simulink library "vmc"  (R2021b)
settings: Solver=VariableStepAuto  StartTime=0.0  StopTime=10.0  RelTol=1e-3
undefined symbols (not defined in the file or in its folder): AVMC_ACCDeltaTqIGain4OVRD_X_kph, AVMC_ACCDeltaTqIGain4OVRD_Y_mps2, AVMC_ACCDeltaTqIGain_X_kph, AVMC_ACCDeltaTqIGain_Y_mps2, AVMC_ACCDeltaTqPGain_X_kph, AVMC_ACCDeltaTqPGain_Y_kph, AVMC_ACCLongSteadyCtrl_X_kph, AVMC_ADSPosGFBDeltaTq_X_kph, AVMC_ADSPosGFBDeltaTq_Y_mps2, AVMC_AggressJerkPCT4AT_X_kph, AVMC_AggressJerkPCT_X_kph, AVMC_AggressLimitPCT4AT_X_kph, AVMC_AggressLimitPCT_X_kph, AVMC_CCLongSteadyCtrl_X_kph, AVMC_DISCDeltaTqIGain_X_kph, AVMC_DISCDeltaTqIGain_Y_mps2, AVMC_DISCDeltaTqPGain_X_kph, AVMC_DISCDeltaTqPGain_Y_kph, AVMC_ESCRegenOut_X_kph, AVMC_ESCRegenOut_Y_Deg, AVMC_ESCRegenOutEnSpd_X_Deg, AVMC_ISOAccLimit_X_mps, AVMC_ISODecLimit_X_mps, AVMC_ISOJerk_X_mps, AVMC_LatESCRegenOut_X_kph, AVMC_LatESCRegenOut_Y_Deg, AVMC_LongAccDeadZone_X_kph, AVMC_LongAccFiltTsforP2_X_Gps, AVMC_MCPresBaseTq_X_bar, AVMC_MSALongSteadyCtrl_X_kph, AVMC_MSAPedalOvrd_X_kph, AVMC_MSASpdBand_X_kph, AVMC_MSATqDownEndTq_X_kph, AVMC_MSATqDownTime_X_kph, AVMC_OPDDisSlideRate_X_Deg, AVMC_OVRD2ActSR2FCMCMD_X_mps2, AVMC_PedalTqRWhlRatio_X_Nm, AVMC_PedalTqRWhlRatio_Y_gps, AVMC_PedalTqRWhlSlipGain_X_rat, AVMC_PedalTqRWhlSlipGain_Y_kph, AVMC_PedalTqRWhSTRGGain_X_deg, AVMC_PedalTqRWhSTRGGain_Y_kph, AVMC_RDCDetectTime_X_kph, AVMC_RDCDetectTime_Y_pct, AVMC_RDCEnSlideRate_X_Deg, AVMC_RearWhlTqRatio_X_Nm, AVMC_RearWhlTqRatio_Y_gps, AVMC_RearWhlTqSlipGain_X_rat, AVMC_RearWhlTqSlipGain_Y_kph, AVMC_RearWhlTqSTRGGain_X_deg, AVMC_RearWhlTqSTRGGain_Y_kph, AVMC_ReqBrkJoinDecSR_X_mps2, AVMC_SoftJerkPCT_X_kph, AVMC_SoftLimitPCT_X_kph, AVMC_StESCYaw_X_kph, AVMC_StESCYaw_Y_Deg, AVMC_StESCYawCom_X_kph, AVMC_StESCYawCom_Y_Gps, AVMC_TMSpdBaseTq_X_rpm, AVMC_VehHoldDecCtrlTime2_X_kph ... (+405)
libraries: hcu_lib x105, simulink x75, tqr x1, simulink_extras x1
(part 13 of 14)

== system vmc/VMC/VMC/Slide Rate  Calculation/4Wheel Calculation/RR Wheel ==
  VVMC_4WheelLongAcc_Gps : Inport
  task_time_s : Inport  Port=2
  VINP_RRRawWhlSpeed_kph : Inport  Port=3
  VTQD_GearActualPosn_enum : Inport  Port=4
  AND4 : Logic  Inputs=3  AllPortsSameDT=off  OutDataTypeStr=boolean
  Abs3 : Abs
  Add : Sum
  Add{3,8,15..16} (4 alike) : Sum  Inputs=+-
  Constant1 : Constant  Value=GRAVITY_G
  Constant11 : Constant  Value=KPH2MPS
  Constant14 : Constant  Value=ONE_PERCENT
  Constant15 : Constant  Value=KVMC_RawWhlSpeedDeadZone_kph
  Constant16 : Constant  Value=ZERO_FLOAT
  Constant17 : Constant  Value=KVMC_RawWhlSpeedDeadZone_kph
  Constant18 : Constant  Value=ONE_FLOAT
  Constant2 : Constant  Value=MPS2KPH
  Constant33 : Constant  Value=KPH2MPS
  Constant34 : Constant  Value=GRAVITY_G
  Constant35 : Constant  Value=KVMC_WhlSpdCalAccTs_c
  Constant42 : Constant  Value=KVMC_WheelSkidAccDev_Gps
  Constant43 : Constant  Value=KVMC_SkidRecVehSpdDev_kph
  Constant44 : Constant  Value=KPH2MPS
  Constant46 : Constant  Value=ENUM_GEARACTUALPOSN_D
  Constant47 : Constant  Value=ENUM_GEARACTUALPOSN_R
  Constant48 : Constant  Value=KVMC_PreVehSpdCalSW_flg
  Constant49 : Constant  Value=KVMC_RRWhlSkidReset_flg
  Constant5 : Constant  Value=KVMC_4WheelEnSkidDetSpd_kph
  Delay{,4..5,12..13,17} (6 alike) : Delay  DelayLength=1
  Divide3 : Product  Inputs=*//
  Divide7 : Product  Inputs=**//
  Equal : RelationalOperator  Operator===  OutDataTypeStr=boolean  RndMeth=Simplest
  Equal1 : RelationalOperator  Operator===  OutDataTypeStr=boolean  RndMeth=Simplest
  FirstOrderFilter3 : hcu_lib/Basic_Blocks/FirstOrderFilter
  OR : Logic  Operator=OR  AllPortsSameDT=off  OutDataTypeStr=boolean
  OR1 : Logic  Operator=OR  AllPortsSameDT=off  OutDataTypeStr=boolean
  OR2 : Logic  Operator=OR  AllPortsSameDT=off  OutDataTypeStr=boolean
  Product : Product
  Product1 : Product  Inputs=3
  Product2 : Product
  Product3 : Product
  Relational Operator14 : RelationalOperator  Operator=>  OutDataTypeStr=boolean  RndMeth=Simplest
  Relational Operator{2,5..6,15} (4 alike) : RelationalOperator  Operator=<=  OutDataTypeStr=boolean  RndMeth=Simplest
  SR_Latch3 : hcu_lib/Basic_Blocks/SR_Latch
  Saturation : Saturate  UpperLimit=KVMC_PredVehSpdLimit_mps  LowerLimit=ZERO_FLOAT
  Switch{,5..6,10} (4 alike) : Switch  Criteria=u2 > Threshold
  VVMC_RRPreVehSpd_kph : Outport
  VVMC_RRWhlSkid_flg : Outport  Port=2
  VVMC_RR4WhlSpdSlideRate_pct : Outport  Port=3
  wires:
  [VINP_RRRawWhlSpeed_kph] -> Add8/1
  Constant49/1 -> AND4/3
  Add8/1 -> Divide7/1
  [task_time_s] -> Divide7/3
  Add15/1 -> Abs3/1
  Relational Operator14/1 -> SR_Latch3/1
  [VVMC_4WheelLongAcc_Gps] -> Add16/2
  [task_time_s] -> FirstOrderFilter3/2
  [VINP_RRRawWhlSpeed_kph] -> Delay4/1
  Constant42/1 -> Relational Operator14/2
  FirstOrderFilter3/1 -> [VVMC_RRWhlCalAcc_Gps]  "VVMC_RRWhlCalAcc_Gps"
  Divide7/1 -> FirstOrderFilter3/1
  Relational Operator15/1 -> AND4/1
  Delay4/1 -> Add8/2
  Delay17/1 -> AND4/2
  [VVMC_RRWhlSkid_flg] -> Delay17/1
  Add16/1 -> Relational Operator14/1
  Delay12/1 -> Add15/1
  Constant43/1 -> Relational Operator15/2
  Delay13/1 -> Add15/2
  Constant33/1 -> Divide7/2
  Constant34/1 -> Divide7/4
  Abs3/1 -> Relational Operator15/1
  SR_Latch3/1 -> [VVMC_RRWhlSkid_flg]  "VVMC_RRWhlSkid_flg"
  [VVMC_RRWhlCalAcc_Gps] -> Add16/1
  Constant35/1 -> FirstOrderFilter3/3
  Constant14/1 -> Divide3/2
  Switch5/1 -> Divide3/3
  Divide3/1 -> Switch6/3  "VVMC_RRCal4WhlSpdSlideRate_pct"
  Switch6/1 -> [VVMC_RR4WhlSpdSlideRate_pct]  "VVMC_RR4WhlSpdSlideRate_pct"
  Constant18/1 -> Switch5/1
  Relational Operator6/1 -> Switch6/2
  [VINP_RRRawWhlSpeed_kph] -> Relational Operator6/1
  Relational Operator5/1 -> Switch5/2
  Constant15/1 -> Relational Operator6/2
  Constant16/1 -> Switch6/1
  Constant17/1 -> Relational Operator5/2
  [VINP_RRRawWhlSpeed_kph] -> Add3/1
  Add3/1 -> Divide3/1
  Product3/1 -> Switch/1
  Constant1/1 -> Product1/2
  Switch10/1 -> [VVMC_RRPreVehSpd_kph]  "VVMC_RRPreVehSpd_kph"
  [VINP_RRRawWhlSpeed_kph] -> Switch10/3
  [VTQD_GearActualPosn_enum] -> Equal/1
  Add/1 -> Product2/1  "VVMC_RRCalPreVehSpd_mps"
  Equal/1 -> OR/1
  Product2/1 -> Switch10/1
  [VVMC_4WheelLongAcc_Gps] -> Product1/1
  Constant11/1 -> Product/2
  Constant44/1 -> Product3/2
  [task_time_s] -> Product1/3
  Switch/1 -> Saturation/1  "VVMC_RRLastPreVehSpd_mps"
  [VVMC_RRPreVehSpd_kph] -> Delay5/1
  Delay/1 -> Product/1
  Constant47/1 -> Equal1/2
  Equal1/1 -> OR/2
  [VTQD_GearActualPosn_enum] -> Equal1/1
  Constant48/1 -> OR1/2
  Constant2/1 -> Product2/2
  OR1/1 -> Switch/2
  Constant46/1 -> Equal/2
  Product1/1 -> Add/1  "VVMC_RRDeltaVehSpd_mps"
  Saturation/1 -> Add/2
  Delay5/1 -> Product3/1
  Product/1 -> Switch/3
  OR/1 -> Switch10/2
  [VVMC_RRWhlSkid_flg] -> OR1/1
  [VINP_RRRawWhlSpeed_kph] -> Delay/1
  [VINP_RRRawWhlSpeed_kph] -> Delay13/1
  [VVMC_RRPreVehSpd_kph] -> Delay12/1
  [VVMC_RRPreVehSpd_kph] -> Add3/2
  [VVMC_RRPreVehSpd_kph] -> Relational Operator5/1
  [VVMC_RRPreVehSpd_kph] -> Switch5/3
  VVMC_4WheelLongAcc_Gps/1 -> [VVMC_4WheelLongAcc_Gps]
  VTQD_GearActualPosn_enum/1 -> [VTQD_GearActualPosn_enum]
  task_time_s/1 -> [task_time_s]
  VINP_RRRawWhlSpeed_kph/1 -> [VINP_RRRawWhlSpeed_kph]
  [VVMC_RRPreVehSpd_kph] -> VVMC_RRPreVehSpd_kph/1
  [VVMC_RRWhlSkid_flg] -> VVMC_RRWhlSkid_flg/1
  [VVMC_RR4WhlSpdSlideRate_pct] -> VVMC_RR4WhlSpdSlideRate_pct/1
  Constant5/1 -> Relational Operator2/2
  [VINP_RRRawWhlSpeed_kph] -> Relational Operator2/1
  Relational Operator2/1 -> OR2/1
  AND4/1 -> OR2/2
  OR2/1 -> SR_Latch3/2  "VVMC_RRWhlSkidReset_flg"

== stateflow chart vmc/VMC/VMC/SpeedArbitration/Feature Arbitration/Feature Arbitration ==
  state FeatureArbitration
    (default) -> (junction 406) : {VVMC_FeatArbitrSta_enum = ENUM_FEATARBITRSTA_INACTIVE;
        |  VVMC_FeatReqSpd_kph = ZERO_FLOAT;}
    FeatureArbitration -> (junction 406)
    (junction 406) -> (junction 409) [order 1] : [VVMC_FeatStaConfirm_enum == ENUM_FEATSTACFM_AEB]
    (junction 406) -> (junction 413) [order 2]
    (junction 409) -> (junction 411) : {VVMC_FeatArbitrSta_enum = ENUM_FEATARBITRSTA_AEB;
        |  VVMC_FeatReqSpd_kph = ZERO_FLOAT}
    (junction 413) -> (junction 415) [order 1] : [VVMC_FeatStaConfirm_enum == ENUM_FEATSTACFM_ACC]
    (junction 413) -> (junction 430) [order 2]
    (junction 415) -> (junction 417) : {VVMC_FeatArbitrSta_enum = ENUM_FEATARBITRSTA_ACC;
        |  VVMC_FeatReqSpd_kph = ZERO_FLOAT}
    (junction 430) -> (junction 431) [order 1] : [VVMC_FeatStaConfirm_enum == ENUM_FEATSTACFM_CC]
    (junction 430) -> (junction 440) [order 2]
    (junction 431) -> (junction 433) : {VVMC_FeatArbitrSta_enum = ENUM_FEATARBITRSTA_CC;
        |  VVMC_FeatReqSpd_kph = VVMC_FeatSetSpdForCalcu_kph}
    (junction 440) -> (junction 441) [order 1] : [VVMC_FeatStaConfirm_enum == ENUM_FEATSTACFM_DISC]
    (junction 440) -> (junction 445) [order 2]
    (junction 441) -> (junction 438) : {VVMC_FeatArbitrSta_enum = ENUM_FEATARBITRSTA_DISC;
        |  VVMC_FeatReqSpd_kph = VDSC_DISCTargetSpd_kph}
    (junction 445) -> (junction 443) [order 1] : [VVMC_FeatStaConfirm_enum == ENUM_FEATSTACFM_MSA]
    (junction 445) -> (junction 449) [order 2]
    (junction 443) -> (junction 444) : {VVMC_FeatArbitrSta_enum = ENUM_FEATARBITRSTA_MSA;
        |  VVMC_FeatReqSpd_kph = VVMC_FeatSetSpdForCalcu_kph}
    (junction 449) -> (junction 450) [order 1] : [VVMC_FeatStaConfirm_enum == ENUM_FEATSTACFM_ACCDISC]
    (junction 450) -> (junction 557) [order 1] : [VVMC_FeatSetSpdForCalcu_kph < VDSC_DISCTargetSpd_kph &&...
        |  !VDSC_PreACC_flg]
    (junction 449) -> (junction 512) [order 2]
    (junction 450) -> (junction 467) [order 2] : {VVMC_FeatArbitrSta_enum = ENUM_FEATARBITRSTA_ACCDISC;
        |  VVMC_FeatReqSpd_kph = VDSC_DISCTargetSpd_kph}
    (junction 557) -> (junction 553) : {VVMC_FeatArbitrSta_enum = ENUM_FEATARBITRSTA_ACC;
        |  VVMC_FeatReqSpd_kph = ZERO_FLOAT}
    (junction 512) -> (junction 514) [order 1] : [VVMC_FeatStaConfirm_enum == ENUM_FEATSTACFM_CCDISC ||...
        |  VVMC_FeatStaConfirm_enum == ENUM_FEATSTACFM_DISCMSA]
    (junction 514) -> (junction 516) [order 1] : [VVMC_FeatSetSpdForCalcu_kph < VDSC_DISCTargetSpd_kph]
    (junction 516) -> (junction 518) [order 1] : [VVMC_FeatStaConfirm_enum == ENUM_FEATSTACFM_CCDISC]
    (junction 512) -> (junction 527) [order 2] : {VVMC_FeatArbitrSta_enum = ENUM_FEATARBITRSTA_INACTIVE;
        |  VVMC_FeatReqSpd_kph = ZERO_FLOAT}
    (junction 514) -> (junction 525) [order 2] : {VVMC_FeatArbitrSta_enum = ENUM_FEATARBITRSTA_DISC;
        |  VVMC_FeatReqSpd_kph = VDSC_DISCTargetSpd_kph}
    (junction 516) -> (junction 522) [order 2] : {VVMC_FeatArbitrSta_enum = ENUM_FEATARBITRSTA_MSA;
        |  VVMC_FeatReqSpd_kph = VVMC_FeatSetSpdForCalcu_kph}
    (junction 518) -> (junction 520) : {VVMC_FeatArbitrSta_enum = ENUM_FEATARBITRSTA_CC;
        |  VVMC_FeatReqSpd_kph = VVMC_FeatSetSpdForCalcu_kph}
  data: VVMC_FeatStaConfirm_enum input uint8; VDSC_DISCTargetSpd_kph input single; VVMC_FeatSetSpdForCalcu_kph input single; VVMC_FeatArbitrSta_enum output uint8; VVMC_FeatReqSpd_kph output single; ENUM_FEATSTACFM_AEB input uint8; ENUM_FEATSTACFM_ACC input uint8; ENUM_FEATSTACFM_CC input uint8; ENUM_FEATSTACFM_DISC input uint8; ENUM_FEATSTACFM_MSA input uint8; ENUM_FEATSTACFM_ACCDISC input uint8; ENUM_FEATSTACFM_CCDISC input uint8; ENUM_FEATSTACFM_DISCMSA input uint8; ENUM_FEATARBITRSTA_INACTIVE input uint8; ENUM_FEATARBITRSTA_AEB input uint8; ENUM_FEATARBITRSTA_ACC input uint8; ENUM_FEATARBITRSTA_CC input uint8; ENUM_FEATARBITRSTA_DISC input uint8; ENUM_FEATARBITRSTA_ACCDISC input uint8; ENUM_FEATARBITRSTA_MSA input uint8; ZERO_FLOAT input single; VDSC_PreACC_flg input

== stateflow chart vmc/VMC/VMC/SPD2ACC/SPD2ACC Active Determination/SPD2ACC Active Determination ==
  state SPD2ACCActiveDetermination
    (default) -> (junction 4) : {VVMC_SPD2ACCAct_flg = FALSE}
    SPD2ACCActiveDetermination -> (junction 4)
    (junction 4) -> (junction 7) [order 1] : [VVMC_FeatArbitrSta_enum == ENUM_FEATARBITRSTA_DISC ||...
        |  VVMC_FeatArbitrSta_enum == ENUM_FEATARBITRSTA_CC ||...
        |  VVMC_FeatArbitrSta_enum == ENUM_FEATARBITRSTA_MSA ||...
        |  VVMC_FeatArbitrSta_enum == ENUM_FEATARBITRSTA_ACCDISC]
    (junction 4) -> (junction 12) [order 2] : {VVMC_SPD2ACCAct_flg = FALSE}
    (junction 7) -> (junction 10) : {VVMC_SPD2ACCAct_flg = TURE}
  data: VVMC_FeatArbitrSta_enum input uint8; VVMC_SPD2ACCAct_flg output boolean; TURE input boolean; FALSE input boolean; ENUM_FEATARBITRSTA_DISC input uint8; ENUM_FEATARBITRSTA_ACCDISC input uint8; ENUM_FEATARBITRSTA_CC input; ENUM_FEATARBITRSTA_MSA input

== stateflow chart vmc/VMC/VMC/MSA function/MSAActivationHandshake/Chart ==
  state MSA_Handshaking
    (default) -> (junction 391) : {VVMC_IntMSACtrlSta_enum = 0;
        |  VVMC_IntMSASpdWar_flg = 0;
        |  VVMC_WaitResetSpdLoop_flg = 0;}
    MSA_Handshaking -> (junction 391) [order 4] : {VVMC_WaitResetSpdLoop_flg = 0;
        |  VVMC_CheckMeterSpdLoop_flg = 0;
        |  VVMC_CheckCmdLoop_flg = 0}
    (junction 391) -> (junction 463) [order 1] : [(VTQD_SpdCtrlMode_enum == 3 ||...
        |  VTQD_SpdCtrlMode_enum == 4) && ...
        |  VVMC_VMCMSACtrlAvail_flg &&... %241026
        |  VTQD_GearActualPosn_enum == ENUM_GEARACTUALPOSN_D]
        | %add20230706
    (junction 463) -> (junction 392) [order 1] : [VTQD_ExternalTqAllow_flg]
    (junction 391) -> (junction 467) [order 2] : {VVMC_IntMSACtrlSta_enum = 0;}
        | %Phase2 VVMC_MSAActive_flg = 0;}
        | %add20230706
    (junction 463) -> (junction 468) [order 2] : {VVMC_IntMSACtrlSta_enum = 5;}
        | %Phase2  VVMC_MSAActive_flg = 0;}
        | %add20230706
    (junction 392) -> (junction 389) : {VVMC_IntMSACtrlSta_enum = 1;}
    MSA_Handshaking -> (junction 389) [order 3] : [VVMC_WaitResetSpdLoop_flg && VTQD_ExternalTqAllow_flg]
        | {VVMC_WaitResetSpdLoop_flg = 0;} %add20230705
    (junction 389) -> (junction 464) [order 1] : [VVMC_DetectSWCSet_flg &&... %241022
        |  VVMC_FeatSetSpdFinal_raw32 > ONE_FLOAT]
    (junction 389) -> (junction 469) [order 2]
    (junction 464) -> (junction 330)
    MSA_Handshaking -> (junction 330) [order 1] : [VVMC_CheckMeterSpdLoop_flg && VTQD_ExternalTqAllow_flg]
        | {VVMC_CheckMeterSpdLoop_flg = 0;}
        | %Phase2 add
    (junction 330) -> (junction 332) [order 1] : [VVMC_FeatSetSpdFinal_raw32 >= KVMC_MSAActiveMetSpdLo_kph &&...
        |  VVMC_FeatSetSpdFinal_raw32 <=  KVMC_MSAActiveMetSpdHi_kph]
    (junction 330) -> (junction 338) [order 2] : {VVMC_IntMSASpdWar_flg = 0;}
    (junction 332) -> (junction 335) : {VVMC_IntMSACtrlSta_enum = 2;}
        | %Phase2 VVMC_MSAActive_flg = 1;}
    (junction 338) -> (junction 339) [order 1] : [VVMC_FeatSetSpdFinal_raw32 > KVMC_MSAActiveMetSpdHi_kph]
    (junction 335) -> (junction 336) [order 1] : [(VVMC_MeterIndSpeedForCalcu_kph - VVMC_FeatSetSpdFinal_raw32)...
        | >= KVMC_CCMSASpdWar_kph]
    (junction 338) -> (junction 334) [order 2] : {VVMC_IntMSACtrlSta_enum = 3;}
    (junction 339) -> (junction 333) : {VVMC_IntMSACtrlSta_enum = 4;}
    (junction 335) -> (junction 346) [order 2] : {VVMC_IntMSASpdWar_flg = 0;}
    (junction 336) -> (junction 345) : {VVMC_IntMSASpdWar_flg = 1;}
    (junction 334) -> (junction 333)
    (junction 333) -> (junction 337) : {VVMC_WaitResetSpdLoop_flg = 1;}
    (junction 346) -> (junction 345)
    (junction 345) -> (junction 342) [order 1] : [(VTQD_SpdCtrlMode_enum != 3 && VTQD_SpdCtrlMode_enum != 4) ||...
        |   VVMC_DetectSWCCANCEL_flg == 1||...
        |  !VTQD_ExternalTqAllow_flg] %Phase2 add20230815
        | %add20230706
    (junction 345) -> (junction 471) [order 2]
    (junction 342) -> (junction 348) : {VVMC_IntMSASpdWar_flg = 0;}
    (junction 471) -> (junction 472) [order 1] : [VVMC_MSAOvrdAllow_flg == 1]
    (junction 471) -> (junction 474) [order 2] : {VVMC_IntMSACtrlSta_enum = 2;}
    (junction 472) -> (junction 473) : {VVMC_IntMSACtrlSta_enum = 7;}
    (junction 474) -> (junction 473)
    (junction 473) -> (junction 347) : {VVMC_CheckMeterSpdLoop_flg = 1;}
    (junction 348) -> (junction 343) [order 1] : [!VTQD_ExternalTqAllow_flg] %Phase2 add20230815
    (junction 348) -> (junction 360) [order 2]
    (junction 343) -> (junction 344) : %Phase2 add20230815
        | {VVMC_IntMSACtrlSta_enum = 5;}
        | %Back to outer first loop.
    MSA_Handshaking -> (junction 360) [order 2] : [VVMC_CheckCmdLoop_flg && VTQD_ExternalTqAllow_flg]
        | {VVMC_CheckCmdLoop_flg = 0;} %Phase2 add 20231003
    (junction 360) -> (junction 350) [order 1] : [(VTQD_SpdCtrlMode_enum != 3 && VTQD_SpdCtrlMode_enum != 4)] %241018 %Phase2 add
    (junction 360) -> (junction 353) [order 2] : %Phase2 {VVMC_MSAActive_flg = 0;
        | {VVMC_IntMSACtrlSta_enum = 1;}
    (junction 350) -> (junction 373) : %Phase2 {VVMC_MSAActive_flg = 0;
        | {VVMC_IntMSACtrlSta_enum = 0;}
        |  %Back to outer first loop.
    (junction 353) -> (junction 354) [order 1] : [VVMC_DetectSWCRes_flg == 1 ||...
        |  VVMC_DetectSWCSet_flg == 1]
        | %Phase2 add
    (junction 353) -> (junction 370) [order 2] : {VVMC_CheckCmdLoop_flg = 1}
        | %Phase2 Modify 20231003
    (junction 354) -> (junction 349) : {VVMC_CheckMeterSpdLoop_flg = 1}
        | %Phase2 add
  MSA_Handshaking -> MSA_Handshaking [order 1] : [!VTQD_ExternalTqAllow_flg || VTQD_GearActualPosn_enum ~= ENUM_GEARACTUALPOSN_D ||...
      |  (VTQD_SpdCtrlMode_enum != 3 && VTQD_SpdCtrlMode_enum != 4) || !VVMC_VMCMSACtrlAvail_flg] %241018
      | %add20240906
  data: VTQD_SpdCtrlMode_enum input uint8; VVMC_IntMSACtrlSta_enum output uint8; VVMC_IntMSASpdWar_flg output boolean; VTQD_ExternalTqAllow_flg input boolean; KVMC_MSAActiveMetSpdHi_kph input single; VVMC_MeterIndSpeedForCalcu_kph input single; KVMC_MSAActiveMetSpdLo_kph input single; VVMC_FeatSetSpdFinal_raw32 input single; KVMC_CCMSASpdWar_kph input single; VVMC_DetectSWCCANCEL_flg input boolean; VVMC_MSAOvrdAllow_flg input; VVMC_CheckMeterSpdLoop_flg local boolean; VVMC_WaitResetSpdLoop_flg local boolean; VVMC_DetectSWCRes_flg input boolean; VVMC_DetectSWCSet_flg input boolean; VVMC_CheckCmdLoop_flg local boolean; ONE_FLOAT parameter; VTQD_GearActualPosn_enum input; ENUM_GEARACTUALPOSN_D parameter; VVMC_VMCMSACtrlAvail_flg input

== stateflow chart vmc/VMC/VMC/CruiseControlFunction/CCActiveDetermination/Chart ==
  state CCActiveDetermination
    (default) -> (junction 360) : {
        |  VVMC_CCCtrlSta_enum = 0;
        |  VVMC_CCSpdWar_flg = 0;
        |  VVMC_SWCResUpLoop_flg = 0;
        |  VVMC_CruzLoopSpdChk_flg = 0;
        |  VVMC_CheckCmdLoop_flg = 0;
        |  }
    CCActiveDetermination -> (junction 360) [order 4] : {VVMC_SWCResUpLoop_flg = 0;
        |  VVMC_CheckCmdLoop_flg = 0;
        |  VVMC_CruzLoopSpdChk_flg = 0;}
    (junction 360) -> (junction 353) [order 1] : [VTQD_SpdCtrlMode_enum == 2 &&...
        |  VVMC_VMCCCCtrlAvail_flg] %241026
    (junction 353) -> (junction 347) [order 1] : [VTQD_ExternalTqAllow_flg]
    (junction 360) -> (junction 343) [order 2] : {VVMC_CCCtrlSta_enum = 0;}
        | %Phase2 VVMC_CruzActive_flg = 0;}
        | %Back to first loop
        | %add20230706
    (junction 353) -> (junction 367) [order 2] : {VVMC_CCCtrlSta_enum = 5;}
        | %Phase2 VVMC_CruzActive_flg = 0;}
        | %Back to first loop
        | %add20230706
    (junction 347) -> (junction 361) : {VVMC_CCCtrlSta_enum = 1;}
    CCActiveDetermination -> (junction 361) [order 3] : [VVMC_SWCResUpLoop_flg && VTQD_ExternalTqAllow_flg]{VVMC_SWCResUpLoop_flg = 0;} %add20230705 %Phase2 modify
    (junction 361) -> (junction 368) [order 1] : [VVMC_FeatSetSpdFinal_raw32 > ONE_FLOAT &&...
        |  VINP_ADASAEBSta_enum ~= ENUM_ADASAEBSTA_ACTIVE]
    (junction 361) -> (junction 374) [order 2] : %Back to first loop
    (junction 368) -> (junction 344)
    CCActiveDetermination -> (junction 344) [order 1] : [VVMC_CruzLoopSpdChk_flg && VTQD_ExternalTqAllow_flg]{VVMC_CruzLoopSpdChk_flg = 0;} %add20230705
    (junction 344) -> (junction 345) [order 1] : [VVMC_FeatSetSpdFinal_raw32 >= KVMC_CCActiveMetSpdLo_kph &&...
        |  VVMC_FeatSetSpdFinal_raw32 <= KVMC_CCActiveMetSpdHi_kph]
    (junction 344) -> (junction 370) [order 2] : {VVMC_CCSpdWar_flg = 0;}
    (junction 345) -> (junction 375) : %Phase 2 {VVMC_CruzActive_flg = 1;
        | {VVMC_CCCtrlSta_enum = 2;}
    (junction 370) -> (junction 371) [order 1] : [VVMC_FeatSetSpdFinal_raw32 < KVMC_CCActiveMetSpdLo_kph]
    (junction 370) -> (junction 348) [order 2] : {VVMC_CCCtrlSta_enum = 4;}
        | %TBD
    (junction 371) -> (junction 346) : {VVMC_CCCtrlSta_enum = 3;}
        | %TBD
    (junction 346) -> (junction 348)
    (junction 348) -> (junction 355) : {VVMC_SWCResUpLoop_flg = 1;}
    (junction 375) -> (junction 349) [order 1] : [(VINP_VehSpeed_kph - VVMC_FeatSetSpdFinal_raw32) >=...
        |  KVMC_CCMSASpdWar_kph]
    (junction 375) -> (junction 356) [order 2] : {VVMC_CCSpdWar_flg = 0;}
    (junction 349) -> (junction 363) : {VVMC_CCSpdWar_flg = 1;}
    (junction 363) -> (junction 356)
    (junction 356) -> (junction 376)
    (junction 376) -> (junction 350) [order 1] : [VVMC_CCPedalOvrd_flg]
    (junction 376) -> (junction 351) [order 2] : {VVMC_CCCtrlSta_enum = 2}
    (junction 350) -> (junction 358) : {VVMC_CCCtrlSta_enum = 7}
    (junction 358) -> (junction 351)
    (junction 351) -> (junction 352)
    (junction 352) -> (junction 354) [order 1] : [ VTQD_SpdCtrlMode_enum != 2 ||...
        |   VVMC_DetectSWCCANCEL_flg ||...
        |   VINP_BrkSwSta_flg ||...
        |   VINP_BrakeSWGPIO_flg  ||...
        |   VINP_ADASAEBSta_enum == ENUM_ADASAEBSTA_ACTIVE] %Phase2 add
    (junction 352) -> (junction 357) [order 2] : {VVMC_CruzLoopSpdChk_flg = 1;}
        | %Phase2 modify
    (junction 354) -> (junction 359) : {VVMC_CCSpdWar_flg = 0;}
    CCActiveDetermination -> (junction 359) [order 2] : [VVMC_CheckCmdLoop_flg && VTQD_ExternalTqAllow_flg]{VVMC_CheckCmdLoop_flg = 0;}
    (junction 359) -> (junction 362) [order 1] : [VTQD_SpdCtrlMode_enum == 2 &&...
        |  !VVMC_DetectSWCCANCEL_flg]
    (junction 359) -> (junction 364) [order 2] : %Phase2 {VVMC_CruzActive_flg = 0;
        | {VVMC_CCCtrlSta_enum = 0;}
        | %Back to first loop
    (junction 362) -> (junction 365) : %Phase 2 {VVMC_CruzActive_flg = 0;
        | {VVMC_CCCtrlSta_enum = 1;
        |  VVMC_SWCSetDownLoop_flg = 1;} %Phase2 add
    (junction 365) -> (junction 432) [order 1] : [VVMC_DetectSWCResUp_flg == 1 ||...
        |  VVMC_DetectSWCSetDown_flg == 1]
        | %Phase2 add
    (junction 365) -> (junction 431) [order 2] : {VVMC_CheckCmdLoop_flg = 1}
    (junction 432) -> (junction 433) : {VVMC_SWCResUpLoop_flg = 1}
        | %Phase2 add
  CCActiveDetermination -> CCActiveDetermination [order 1] : [!VTQD_ExternalTqAllow_flg || VTQD_GearActualPosn_enum ~= ENUM_GEARACTUALPOSN_D || !VTQD_ExtDoorAllow_flg || !VVMC_VMCCCCtrlAvail_flg]
      | %add20240918
  data: VVMC_CCCtrlSta_enum output uint8; VTQD_SpdCtrlMode_enum input uint8; VVMC_CCSpdWar_flg output boolean; VTQD_ExternalTqAllow_flg input boolean; VVMC_DetectSWCSetDown_flg input boolean; KVMC_CCActiveMetSpdHi_kph input single; VINP_VehSpeed_kph input single; KVMC_CCActiveMetSpdLo_kph input single; VVMC_FeatSetSpdFinal_raw32 input single; KVMC_CCMSASpdWar_kph input single; VINP_BrakeSWGPIO_flg input boolean; VVMC_DetectSWCCANCEL_flg input boolean; VINP_BrkSwSta_flg input boolean; VVMC_DetectSWCResUp_flg input boolean; VVMC_CruzLoopSpdChk_flg local boolean; VVMC_SWCSetDownLoop_flg local boolean; VINP_ADASAEBSta_enum input uint8; ENUM_ADASAEBSTA_ACTIVE input uint8; VVMC_CCPedalOvrd_flg input boolean; VTQD_GearActualPosn_enum input uint8; ENUM_GEARACTUALPOSN_D input uint8; VVMC_CheckCmdLoop_flg local boolean; VVMC_SWCResUpLoop_flg local boolean; ONE_FLOAT parameter; VTQD_ExtDoorAllow_flg input; VVMC_VMCCCCtrlAvail_flg input

== stateflow chart vmc/VMC/VMC/ACC_Function/ACC Torque Source Determination/TimeGapJudgement ==
  state TimeGapJudgement
    (default) -> (junction 11) : {VVMC_TimeGapJudge_flag = FALSE}
    TimeGapJudgement -> (junction 11)
    (junction 11) -> (junction 71) [order 1] : [(VINP_VehSpeed_kph * KPH2MPS) > ZERO_FLOAT]
    (junction 11) -> (junction 33) [order 2] : {VVMC_TimeGapJudge_flag = FALSE;
        |  VVMC_TimeGapCalcu_s = KVMC_TimeGapMax_s}
    (junction 71) -> (junction 24) : {VVMC_TimeGapCalcu_s = VINP_ACCObjDist_m / (VINP_VehSpeed_kph * KPH2MPS)}
    (junction 24) -> (junction 29) [order 1] : [VINP_TimeGapLevel_enum == ENUM_TIMEGAPLEVEL_LEVEL1]
    (junction 29) -> (junction 27) [order 1] : [VVMC_TimeGapCalcu_s <= KVMC_TimeGapBandLv1_s]
    (junction 24) -> (junction 35) [order 2]
    (junction 29) -> (junction 44) [order 2] : {VVMC_TimeGapJudge_flag = FALSE}
    (junction 27) -> (junction 31) : {VVMC_TimeGapJudge_flag = TRUE}
    (junction 35) -> (junction 38) [order 1] : [VINP_TimeGapLevel_enum == ENUM_TIMEGAPLEVEL_LEVEL2]
    (junction 38) -> (junction 42) [order 1] : [VVMC_TimeGapCalcu_s <= KVMC_TimeGapBandLv2_s]
    (junction 35) -> (junction 56) [order 2]
    (junction 38) -> (junction 46) [order 2] : {VVMC_TimeGapJudge_flag = FALSE}
    (junction 42) -> (junction 40) : {VVMC_TimeGapJudge_flag = TRUE}
    (junction 56) -> (junction 49) [order 1] : [VINP_TimeGapLevel_enum == ENUM_TIMEGAPLEVEL_LEVEL3]
    (junction 49) -> (junction 50) [order 1] : [VVMC_TimeGapCalcu_s <= KVMC_TimeGapBandLv3_s]
    (junction 56) -> (junction 59) [order 2]
    (junction 49) -> (junction 48) [order 2] : {VVMC_TimeGapJudge_flag = FALSE}
    (junction 50) -> (junction 53) : {VVMC_TimeGapJudge_flag = TRUE}
    (junction 59) -> (junction 65) [order 1] : [VINP_TimeGapLevel_enum == ENUM_TIMEGAPLEVEL_LEVEL4]
    (junction 65) -> (junction 64) [order 1] : [VVMC_TimeGapCalcu_s <= KVMC_TimeGapBandLv4_s]
    (junction 59) -> (junction 68) [order 2] : {VVMC_TimeGapJudge_flag = FALSE}
    (junction 65) -> (junction 66) [order 2] : {VVMC_TimeGapJudge_flag = FALSE}
    (junction 64) -> (junction 58) : {VVMC_TimeGapJudge_flag = TRUE}
  data: VINP_ACCObjDist_m input single; VINP_VehSpeed_kph input single; KPH2MPS input single; VINP_TimeGapLevel_enum input uint8; VVMC_TimeGapJudge_flag output boolean; ENUM_TIMEGAPLEVEL_LEVEL1 input uint8; KVMC_TimeGapBandLv1_s input single; ENUM_TIMEGAPLEVEL_LEVEL2 input uint8; KVMC_TimeGapBandLv2_s input single; ENUM_TIMEGAPLEVEL_LEVEL3 input uint8; KVMC_TimeGapBandLv3_s input single; ENUM_TIMEGAPLEVEL_LEVEL4 input uint8; KVMC_TimeGapBandLv4_s input single; TRUE input boolean; FALSE input boolean; ZERO_FLOAT input single; KVMC_TimeGapMax_s input single; VVMC_TimeGapCalcu_s output single

== stateflow chart vmc/VMC/VMC/SPD2ACC/VVMC_DISReqAcc_mps2/CMDRepeat ==
  state CMDCycleTime
    (default) -> (junction 4) : {VVMC_CMDCount_enum = ZERO_INT}
    CMDCycleTime -> (junction 4)
    (junction 4) -> (junction 8) [order 1] : [VVMC_SPD2ACCAct_flg == TRUE &&...
        | (VVMC_DISCReqAccAftLim_mps2 > ZERO_FLOAT ||...
        |  VVMC_DISCReqAccAftLim_mps2 < ZERO_FLOAT)]
    (junction 8) -> (junction 13) [order 1] : [VVMC_CMDCount_enum == ZERO_INT ||...
        |  KVMC_CMDRepeatTime_enum == ZERO_INT]
    (junction 13) -> (junction 31) [order 1] : [KVMC_CMDRepeatTime_enum == ZERO_INT]
    (junction 4) -> (junction 21) [order 2] : {VVMC_DISCReqAccAftRepeat_mps2 = ZERO_FLOAT;
        |  VVMC_CMDCount_enum = ZERO_INT}
    (junction 8) -> (junction 11) [order 2]
    (junction 13) -> (junction 15) [order 2] : {VVMC_DISCReqAccAftRepeat_mps2 = VVMC_DISCReqAccAftLim_mps2;
        |  VVMC_CMDCount_enum++}
    (junction 31) -> (junction 33) : {VVMC_DISCReqAccAftRepeat_mps2 = VVMC_DISCReqAccAftLim_mps2;}
    (junction 11) -> (junction 17) [order 1] : [VVMC_CMDCount_enum < KVMC_CMDRepeatTime_enum]
    (junction 11) -> (junction 23) [order 2] : {VVMC_CMDCount_enum = ZERO_INT}
    (junction 17) -> (junction 19) : {VVMC_CMDCount_enum++}
  data: VVMC_DISCReqAccAftLim_mps2 input single; TRUE input; ZERO_FLOAT input; VVMC_CMDCount_enum local uint8; VVMC_DISCReqAccAftRepeat_mps2 output single; ZERO_INT input uint8; KVMC_CMDRepeatTime_enum input uint8; VVMC_SPD2ACCAct_flg input

== stateflow chart vmc/VMC/VMC/SPD2ACC/VVMC_DISReqAcc_mps2/ConstantSpeedControl1 ==
  state ConstantSpeedControl
    (default) -> (junction 2) : {SpdCtrlFlag = 0;
        |  ReqAccel = 0}
    ConstantSpeedControl -> (junction 2)
    (junction 2) -> (junction 6) [order 1] : [DeltaSpeed >= KVMC_SpdCtrlEnBand_kph && SpdCtrlFlag == 0 && VVMC_ACCSpdCtrl_flg]
    (junction 2) -> (junction 16) [order 2]
    (junction 6) -> (junction 8) : {SpdCtrlFlag = 1;
        |  ReqAccel = MINUSONE_FLOAT * KVMC_SpdCtrlReqAccel_mps2}
    (junction 16) -> (junction 15) [order 1] : [DeltaSpeed <= MINUSONE_FLOAT * KVMC_SpdCtrlEnBand_kph && SpdCtrlFlag == 0 && VVMC_ACCSpdCtrl_flg]
    (junction 16) -> (junction 20) [order 2]
    (junction 15) -> (junction 12) : {SpdCtrlFlag = 1;
        |  ReqAccel = KVMC_SpdCtrlReqAccel_mps2}
    (junction 20) -> (junction 18) [order 1] : [VVMC_ACCSpdCtrl_flg && SpdCtrlFlag == 1]
    (junction 18) -> (junction 24) [order 1] : [ReqAccel > ZERO_FLOAT]
    (junction 24) -> (junction 26) [order 1] : [DeltaSpeed >= KVMC_SpdCtrlDisBand_kph]
    (junction 20) -> (junction 42) [order 2] : {SpdCtrlFlag = 0;
        |  ReqAccel = ZERO_FLOAT}
    (junction 18) -> (junction 40) [order 2]
    (junction 24) -> (junction 30) [order 2] : {SpdCtrlFlag = 1;
        |  ReqAccel = KVMC_SpdCtrlReqAccel_mps2}
    (junction 26) -> (junction 28) : {SpdCtrlFlag = 0;
        |  ReqAccel = ZERO_FLOAT}
    (junction 40) -> (junction 37) [order 1] : [ReqAccel < ZERO_FLOAT]
    (junction 37) -> (junction 33) [order 1] : [DeltaSpeed <= MINUSONE_FLOAT * KVMC_SpdCtrlDisBand_kph]
    (junction 40) -> (junction 49) [order 2]
    (junction 37) -> (junction 35) [order 2] : {SpdCtrlFlag = 1;
        |  ReqAccel = MINUSONE_FLOAT * KVMC_SpdCtrlReqAccel_mps2}
    (junction 33) -> (junction 38) : {SpdCtrlFlag = 0;
        |  ReqAccel = ZERO_FLOAT}
  data: DeltaSpeed input single; SpdCtrlFlag local boolean; ReqAccel output single; KVMC_SpdCtrlEnBand_kph input single; KVMC_SpdCtrlDisBand_kph input single; MINUSONE_FLOAT input single; KVMC_SpdCtrlReqAccel_mps2 input single; ZERO_FLOAT input single; VVMC_ACCSpdCtrl_flg input

== stateflow chart vmc/VMC/VMC/Scheduler ==
  state Scheduler
    (default) -> (junction 3) : {counter = 0;}
    Scheduler -> (junction 3) : {counter++}
    (junction 3) -> (junction 5) [order 1] : [counter%%2 == 0]
    (junction 3) -> (junction 11) [order 2]
    (junction 5) -> (junction 7) : {Trigger_10ms_1;
        |  counter = 0;}
    (junction 7) -> (junction 11)
  data: counter local uint8
  events: Trigger_10ms_1 output FUNCTION_CALL_EVENT

== stateflow chart vmc/VMC/VMC/SafetyControl/LatAccRollingAverage/RollingAverage ==
  state LatAccelRollingAverage
    (default) -> (junction 2) : {VVMC_RollAveCount_enum = ONE_INT}
    LatAccelRollingAverage -> (junction 2)
    (junction 2) -> (junction 3) : {VVMC_LatAccRollAveRaw_Gps = ZERO_FLOAT}
    (junction 3) -> (junction 100) [order 1] : [VVMC_RollAveCount_enum < KVMC_LatAccRollAveLevel_enum]
    (junction 3) -> (junction 37) [order 2]
    (junction 100) -> (junction 5) : {% Memory
        |  VVMC_Memory_raw32[VVMC_RollAveCount_enum] = VINP_LatAccel_Gps;
        |
        |  % Memory Shift Counter
        |  VVMC_ShiftCount_enum = ONE_INT}
    (junction 5) -> (junction 7) [order 2]
    (junction 5) -> (junction 6) [order 1] : [VVMC_ShiftCount_enum <= VVMC_RollAveCount_enum]
    (junction 7) -> (junction 8) : {% Rolling Average
        |  VVMC_LatAccRollAveRaw_Gps = VVMC_LatAccRollAveRaw_Gps / VVMC_RollAveCount_enum;
        |
        |  % Rolling Average Counter
        |  VVMC_RollAveCount_enum++}
    (junction 35) -> (junction 5) : {VVMC_ShiftCount_enum++}
    (junction 6) -> (junction 36) : {% Rolling Average Sum
        |  VVMC_LatAccRollAveRaw_Gps = VVMC_LatAccRollAveRaw_Gps + VVMC_Memory_raw32[VVMC_ShiftCount_enum];
        |  }
    (junction 36) -> (junction 35)
    (junction 37) -> (junction 76) [order 1] : [VVMC_RollAveCount_enum == KVMC_LatAccRollAveLevel_enum]
    (junction 76) -> (junction 47)
    (junction 37) -> (junction 60) [order 2]
    (junction 78) -> (junction 76)
    (junction 47) -> (junction 30) : {% Memory
        |  VVMC_Memory_raw32[VVMC_RollAveCount_enum] = VINP_LatAccel_Gps;
        |
        |  % Memory Shift Counter
        |  VVMC_ShiftCount_enum = ONE_INT;
        | }
    (junction 60) -> (junction 62) [order 1] : [VVMC_RollAveCount_enum > KVMC_LatAccRollAveLevel_enum]
    (junction 60) -> (junction 39) [order 2]
    (junction 62) -> (junction 66) : {VVMC_MemoryShiftCount_enum = ONE_INT}
    (junction 30) -> (junction 48) [order 2]
    (junction 30) -> (junction 22) [order 1] : [VVMC_ShiftCount_enum <= VVMC_RollAveCount_enum]
    (junction 48) -> (junction 45) : {% Rolling Average
        |  VVMC_LatAccRollAveRaw_Gps = VVMC_LatAccRollAveRaw_Gps / VVMC_RollAveCount_enum;
        |
        |  % Memory Shift Counter
        |  VVMC_ShiftCount_enum = ONE_INT}
    (junction 14) -> (junction 30) : {VVMC_ShiftCount_enum++}
    (junction 22) -> (junction 25) : {% Rolling Average Sum
        |  VVMC_LatAccRollAveRaw_Gps = VVMC_LatAccRollAveRaw_Gps + VVMC_Memory_raw32[VVMC_ShiftCount_enum]}
    (junction 66) -> (junction 82) [order 2]
    (junction 66) -> (junction 69) [order 1] : [VVMC_MemoryShiftCount_enum < VVMC_RollAveCount_enum]
    (junction 82) -> (junction 80) : {VVMC_RollAveCount_enum = KVMC_LatAccRollAveLevel_enum}
    (junction 73) -> (junction 66) : {VVMC_MemoryShiftCount_enum++}
    (junction 69) -> (junction 71) : {VVMC_Memory_raw32[VVMC_MemoryShiftCount_enum] =...
        |  VVMC_Memory_raw32[VVMC_RollAveCount_enum - KVMC_LatAccRollAveLevel_enum + VVMC_MemoryShiftCount_enum]}
    (junction 25) -> (junction 14)
    (junction 71) -> (junction 73)
    (junction 80) -> (junction 78)
    (junction 45) -> (junction 39) [order 2]
    (junction 45) -> (junction 15) [order 1] : [VVMC_ShiftCount_enum < VVMC_RollAveCount_enum]
    (junction 41) -> (junction 45) : { VVMC_ShiftCount_enum++}
    (junction 15) -> (junction 38) : {% Gy Memory Shift
        |  VVMC_Memory_raw32[VVMC_ShiftCount_enum] = VVMC_Memory_raw32[VVMC_ShiftCount_enum + ONE_INT]}
    (junction 38) -> (junction 41)
  data: KVMC_LatAccRollAveLevel_enum input uint8; VVMC_ShiftCount_enum local uint8; VVMC_RollAveCount_enum local uint8; VVMC_Memory_raw32 local single size=256; ZERO_FLOAT input single; ONE_INT input uint8; VINP_LatAccel_Gps input single; VVMC_MemoryShiftCount_enum local uint8; VVMC_LatAccRollAveRaw_Gps output single

== stateflow chart vmc/VMC/VMC/FeatureSetSpeed/SpeedDetermination ==
  state SpeedDetermination
    (default) -> (junction 9) : {VVMC_FeatSetSpdFinal_raw32 = ZERO_FLOAT}
    SpeedDetermination -> (junction 9)
    (junction 9) -> (junction 14) [order 1] : [VVMC_APPSpdLimit_flg == ENUM_APPSPDLIMIT_ON]
    (junction 14) -> (junction 16) [order 1] : [VTQD_SpdCtrlSta_flg == ENUM_SCPCRLSTA_ON]
    (junction 9) -> (junction 22) [order 2]
    (junction 14) -> (junction 20) [order 2] : {VVMC_FeatSetSpdFinal_raw32 = VVMC_APPSpdLimit_kph}
    (junction 16) -> (junction 18) : {VVMC_FeatSetSpdFinal_raw32 =...
        |  min(VVMC_APPSpdLimit_kph, VTQD_SetSpd_kph)}
    (junction 22) -> (junction 24) [order 1] : [VTQD_SpdCtrlSta_flg == ENUM_SCPCRLSTA_ON]
    (junction 22) -> (junction 28) [order 2] : {VVMC_FeatSetSpdFinal_raw32 = ZERO_FLOAT}
    (junction 24) -> (junction 26) : {VVMC_FeatSetSpdFinal_raw32 = VTQD_SetSpd_kph}
  data: VVMC_APPSpdLimit_flg input boolean; VTQD_SpdCtrlSta_flg input boolean; VVMC_APPSpdLimit_kph input single; VTQD_SetSpd_kph input single; ENUM_SCPCRLSTA_ON input uint8; ENUM_APPSPDLIMIT_ON input uint8; VVMC_FeatSetSpdFinal_raw32 output single; ZERO_FLOAT input single

== stateflow chart vmc/VMC/VMC/IMU/IMU sensing result /RollingAverage1 ==
  state RollingAverage
    (default) -> (junction 2) : {VVMC_RollAveCount_enum = ONE_INT}
    RollingAverage -> (junction 2)
    (junction 2) -> (junction 3) : {VVMC_RollAve_raw32 = ZERO_FLOAT}
    (junction 3) -> (junction 100) [order 1] : [VVMC_RollAveCount_enum < KVMC_RollAveLevel_enum]
    (junction 3) -> (junction 37) [order 2]
    (junction 100) -> (junction 5) : {% Memory
        |  VVMC_Memory_raw32[VVMC_RollAveCount_enum] = VINP_INPData_raw32;
        |
        |  % Memory Shift Counter
        |  VVMC_ShiftCount_enum = ONE_INT}
    (junction 5) -> (junction 7) [order 2]
    (junction 5) -> (junction 6) [order 1] : [VVMC_ShiftCount_enum <= VVMC_RollAveCount_enum]
    (junction 7) -> (junction 8) : {% Rolling Average
        |  VVMC_RollAve_raw32 = VVMC_RollAve_raw32 / VVMC_RollAveCount_enum;
        |
        |  % Rolling Average Counter
        |  VVMC_RollAveCount_enum++}
    (junction 35) -> (junction 5) : {VVMC_ShiftCount_enum++}
    (junction 6) -> (junction 36) : {% Rolling Average Sum
        |  VVMC_RollAve_raw32 = VVMC_RollAve_raw32 + VVMC_Memory_raw32[VVMC_ShiftCount_enum];
        |  }
    (junction 36) -> (junction 35)
    (junction 37) -> (junction 76) [order 1] : [VVMC_RollAveCount_enum == KVMC_RollAveLevel_enum]
    (junction 76) -> (junction 47)
    (junction 37) -> (junction 60) [order 2]
    (junction 78) -> (junction 76)
    (junction 47) -> (junction 30) : {% Memory
        |  VVMC_Memory_raw32[VVMC_RollAveCount_enum] = VINP_INPData_raw32;
        |
        |  % Memory Shift Counter
        |  VVMC_ShiftCount_enum = ONE_INT;
        | }
    (junction 60) -> (junction 62) [order 1] : [VVMC_RollAveCount_enum > KVMC_RollAveLevel_enum]
    (junction 60) -> (junction 39) [order 2]
    (junction 62) -> (junction 66) : {VVMC_MemoryShiftCount_enum = ONE_INT}
    (junction 30) -> (junction 48) [order 2]
    (junction 30) -> (junction 22) [order 1] : [VVMC_ShiftCount_enum <= VVMC_RollAveCount_enum]
    (junction 48) -> (junction 45) : {% Rolling Average
        |  VVMC_RollAve_raw32 = VVMC_RollAve_raw32 / VVMC_RollAveCount_enum;
        |
        |  % Memory Shift Counter
        |  VVMC_ShiftCount_enum = ONE_INT}
    (junction 14) -> (junction 30) : {VVMC_ShiftCount_enum++}
    (junction 22) -> (junction 25) : {% Rolling Average Sum
        |  VVMC_RollAve_raw32 = VVMC_RollAve_raw32 + VVMC_Memory_raw32[VVMC_ShiftCount_enum]}
    (junction 66) -> (junction 82) [order 2]
    (junction 66) -> (junction 69) [order 1] : [VVMC_MemoryShiftCount_enum < VVMC_RollAveCount_enum]
    (junction 82) -> (junction 80) : {VVMC_RollAveCount_enum = KVMC_RollAveLevel_enum}
    (junction 73) -> (junction 66) : {VVMC_MemoryShiftCount_enum++}
    (junction 69) -> (junction 71) : {VVMC_Memory_raw32[VVMC_MemoryShiftCount_enum] =...
        |  VVMC_Memory_raw32[VVMC_RollAveCount_enum - KVMC_RollAveLevel_enum + VVMC_MemoryShiftCount_enum]}
    (junction 25) -> (junction 14)
    (junction 71) -> (junction 73)
    (junction 80) -> (junction 78)
    (junction 45) -> (junction 39) [order 2]
    (junction 45) -> (junction 15) [order 1] : [VVMC_ShiftCount_enum < VVMC_RollAveCount_enum]
    (junction 41) -> (junction 45) : { VVMC_ShiftCount_enum++}
    (junction 15) -> (junction 38) : {% Gy Memory Shift
        |  VVMC_Memory_raw32[VVMC_ShiftCount_enum] = VVMC_Memory_raw32[VVMC_ShiftCount_enum + ONE_INT]}
    (junction 38) -> (junction 41)
  data: KVMC_RollAveLevel_enum input uint8; VVMC_ShiftCount_enum local uint8; VVMC_RollAveCount_enum local uint8; VVMC_Memory_raw32 local single size=256; ZERO_FLOAT input single; ONE_INT input uint8; VVMC_RollAve_raw32 output single; VINP_INPData_raw32 input single; VVMC_MemoryShiftCount_enum local uint8

== stateflow chart vmc/VMC/VMC/IMU/IMU sensing result /RollingAverage2 ==
  state RollingAverage
    (default) -> (junction 2) : {VVMC_RollAveCount_enum = ONE_INT}
    RollingAverage -> (junction 2)
    (junction 2) -> (junction 3) : {VVMC_RollAve_raw32 = ZERO_FLOAT}
    (junction 3) -> (junction 100) [order 1] : [VVMC_RollAveCount_enum < KVMC_RollAveLevel_enum]
    (junction 3) -> (junction 37) [order 2]
    (junction 100) -> (junction 5) : {% Memory
        |  VVMC_Memory_raw32[VVMC_RollAveCount_enum] = VINP_INPData_raw32;
        |
        |  % Memory Shift Counter
        |  VVMC_ShiftCount_enum = ONE_INT}
    (junction 5) -> (junction 7) [order 2]
    (junction 5) -> (junction 6) [order 1] : [VVMC_ShiftCount_enum <= VVMC_RollAveCount_enum]
    (junction 7) -> (junction 8) : {% Rolling Average
        |  VVMC_RollAve_raw32 = VVMC_RollAve_raw32 / VVMC_RollAveCount_enum;
        |
        |  % Rolling Average Counter
        |  VVMC_RollAveCount_enum++}
    (junction 35) -> (junction 5) : {VVMC_ShiftCount_enum++}
    (junction 6) -> (junction 36) : {% Rolling Average Sum
        |  VVMC_RollAve_raw32 = VVMC_RollAve_raw32 + VVMC_Memory_raw32[VVMC_ShiftCount_enum];
        |  }
    (junction 36) -> (junction 35)
    (junction 37) -> (junction 76) [order 1] : [VVMC_RollAveCount_enum == KVMC_RollAveLevel_enum]
    (junction 76) -> (junction 47)
    (junction 37) -> (junction 60) [order 2]
    (junction 78) -> (junction 76)
    (junction 47) -> (junction 30) : {% Memory
        |  VVMC_Memory_raw32[VVMC_RollAveCount_enum] = VINP_INPData_raw32;
        |
        |  % Memory Shift Counter
        |  VVMC_ShiftCount_enum = ONE_INT;
        | }
    (junction 60) -> (junction 62) [order 1] : [VVMC_RollAveCount_enum > KVMC_RollAveLevel_enum]
    (junction 60) -> (junction 39) [order 2]
    (junction 62) -> (junction 66) : {VVMC_MemoryShiftCount_enum = ONE_INT}
    (junction 30) -> (junction 48) [order 2]
    (junction 30) -> (junction 22) [order 1] : [VVMC_ShiftCount_enum <= VVMC_RollAveCount_enum]
    (junction 48) -> (junction 45) : {% Rolling Average
        |  VVMC_RollAve_raw32 = VVMC_RollAve_raw32 / VVMC_RollAveCount_enum;
        |
        |  % Memory Shift Counter
        |  VVMC_ShiftCount_enum = ONE_INT}
    (junction 14) -> (junction 30) : {VVMC_ShiftCount_enum++}
    (junction 22) -> (junction 25) : {% Rolling Average Sum
        |  VVMC_RollAve_raw32 = VVMC_RollAve_raw32 + VVMC_Memory_raw32[VVMC_ShiftCount_enum]}
    (junction 66) -> (junction 82) [order 2]
    (junction 66) -> (junction 69) [order 1] : [VVMC_MemoryShiftCount_enum < VVMC_RollAveCount_enum]
    (junction 82) -> (junction 80) : {VVMC_RollAveCount_enum = KVMC_RollAveLevel_enum}
    (junction 73) -> (junction 66) : {VVMC_MemoryShiftCount_enum++}
    (junction 69) -> (junction 71) : {VVMC_Memory_raw32[VVMC_MemoryShiftCount_enum] =...
        |  VVMC_Memory_raw32[VVMC_RollAveCount_enum - KVMC_RollAveLevel_enum + VVMC_MemoryShiftCount_enum]}
    (junction 25) -> (junction 14)
    (junction 71) -> (junction 73)
    (junction 80) -> (junction 78)
    (junction 45) -> (junction 39) [order 2]
    (junction 45) -> (junction 15) [order 1] : [VVMC_ShiftCount_enum < VVMC_RollAveCount_enum]
    (junction 41) -> (junction 45) : { VVMC_ShiftCount_enum++}
    (junction 15) -> (junction 38) : {% Gy Memory Shift
        |  VVMC_Memory_raw32[VVMC_ShiftCount_enum] = VVMC_Memory_raw32[VVMC_ShiftCount_enum + ONE_INT]}
    (junction 38) -> (junction 41)
  data: KVMC_RollAveLevel_enum input uint8; VVMC_ShiftCount_enum local uint8; VVMC_RollAveCount_enum local uint8; VVMC_Memory_raw32 local single size=256; ZERO_FLOAT input single; ONE_INT input uint8; VVMC_RollAve_raw32 output single; VINP_INPData_raw32 input single; VVMC_MemoryShiftCount_enum local uint8

== stateflow chart vmc/VMC/VMC/IMU/IMU sensing result /RollingAverage3 ==
  state RollingAverage
    (default) -> (junction 2) : {VVMC_RollAveCount_enum = ONE_INT}
    RollingAverage -> (junction 2)
    (junction 2) -> (junction 3) : {VVMC_RollAve_raw32 = ZERO_FLOAT}
    (junction 3) -> (junction 100) [order 1] : [VVMC_RollAveCount_enum < KVMC_RollAveLevel_enum]
    (junction 3) -> (junction 37) [order 2]
    (junction 100) -> (junction 5) : {% Memory
        |  VVMC_Memory_raw32[VVMC_RollAveCount_enum] = VINP_INPData_raw32;
        |
        |  % Memory Shift Counter
        |  VVMC_ShiftCount_enum = ONE_INT}
    (junction 5) -> (junction 7) [order 2]
    (junction 5) -> (junction 6) [order 1] : [VVMC_ShiftCount_enum <= VVMC_RollAveCount_enum]
    (junction 7) -> (junction 8) : {% Rolling Average
        |  VVMC_RollAve_raw32 = VVMC_RollAve_raw32 / VVMC_RollAveCount_enum;
        |
        |  % Rolling Average Counter
        |  VVMC_RollAveCount_enum++}
    (junction 35) -> (junction 5) : {VVMC_ShiftCount_enum++}
    (junction 6) -> (junction 36) : {% Rolling Average Sum
        |  VVMC_RollAve_raw32 = VVMC_RollAve_raw32 + VVMC_Memory_raw32[VVMC_ShiftCount_enum];
        |  }
    (junction 36) -> (junction 35)
    (junction 37) -> (junction 76) [order 1] : [VVMC_RollAveCount_enum == KVMC_RollAveLevel_enum]
    (junction 76) -> (junction 47)
    (junction 37) -> (junction 60) [order 2]
    (junction 78) -> (junction 76)
    (junction 47) -> (junction 30) : {% Memory
        |  VVMC_Memory_raw32[VVMC_RollAveCount_enum] = VINP_INPData_raw32;
        |
        |  % Memory Shift Counter
        |  VVMC_ShiftCount_enum = ONE_INT;
        | }
    (junction 60) -> (junction 62) [order 1] : [VVMC_RollAveCount_enum > KVMC_RollAveLevel_enum]
    (junction 60) -> (junction 39) [order 2]
    (junction 62) -> (junction 66) : {VVMC_MemoryShiftCount_enum = ONE_INT}
    (junction 30) -> (junction 48) [order 2]
    (junction 30) -> (junction 22) [order 1] : [VVMC_ShiftCount_enum <= VVMC_RollAveCount_enum]
    (junction 48) -> (junction 45) : {% Rolling Average
        |  VVMC_RollAve_raw32 = VVMC_RollAve_raw32 / VVMC_RollAveCount_enum;
        |
        |  % Memory Shift Counter
        |  VVMC_ShiftCount_enum = ONE_INT}
    (junction 14) -> (junction 30) : {VVMC_ShiftCount_enum++}
    (junction 22) -> (junction 25) : {% Rolling Average Sum
        |  VVMC_RollAve_raw32 = VVMC_RollAve_raw32 + VVMC_Memory_raw32[VVMC_ShiftCount_enum]}
    (junction 66) -> (junction 82) [order 2]
    (junction 66) -> (junction 69) [order 1] : [VVMC_MemoryShiftCount_enum < VVMC_RollAveCount_enum]
    (junction 82) -> (junction 80) : {VVMC_RollAveCount_enum = KVMC_RollAveLevel_enum}
    (junction 73) -> (junction 66) : {VVMC_MemoryShiftCount_enum++}
    (junction 69) -> (junction 71) : {VVMC_Memory_raw32[VVMC_MemoryShiftCount_enum] =...
        |  VVMC_Memory_raw32[VVMC_RollAveCount_enum - KVMC_RollAveLevel_enum + VVMC_MemoryShiftCount_enum]}
    (junction 25) -> (junction 14)
    (junction 71) -> (junction 73)
    (junction 80) -> (junction 78)
    (junction 45) -> (junction 39) [order 2]
    (junction 45) -> (junction 15) [order 1] : [VVMC_ShiftCount_enum < VVMC_RollAveCount_enum]
    (junction 41) -> (junction 45) : { VVMC_ShiftCount_enum++}
    (junction 15) -> (junction 38) : {% Gy Memory Shift
        |  VVMC_Memory_raw32[VVMC_ShiftCount_enum] = VVMC_Memory_raw32[VVMC_ShiftCount_enum + ONE_INT]}
    (junction 38) -> (junction 41)
  data: KVMC_RollAveLevel_enum input uint8; VVMC_ShiftCount_enum local uint8; VVMC_RollAveCount_enum local uint8; VVMC_Memory_raw32 local single size=256; ZERO_FLOAT input single; ONE_INT input uint8; VVMC_RollAve_raw32 output single; VINP_INPData_raw32 input single; VVMC_MemoryShiftCount_enum local uint8

== stateflow chart vmc/VMC/VMC/SafetyControl/VehSpdRollingAverage/RollingAverage ==
  state LatAccelRollingAverage
    (default) -> (junction 2) : {VVMC_RollAveCount_enum = ONE_INT}
    LatAccelRollingAverage -> (junction 2)
    (junction 2) -> (junction 3) : {VVMC_VehSpdRollAveRaw_kph = ZERO_FLOAT}
    (junction 3) -> (junction 100) [order 1] : [VVMC_RollAveCount_enum < KVMC_VehSpdRollAveLevel_enum]
    (junction 3) -> (junction 37) [order 2]
    (junction 100) -> (junction 5) : {% Memory
        |  VVMC_Memory_raw32[VVMC_RollAveCount_enum] = VINP_VehSpeed_kph;
        |
        |  % Memory Shift Counter
        |  VVMC_ShiftCount_enum = ONE_INT}
    (junction 5) -> (junction 7) [order 2]
    (junction 5) -> (junction 6) [order 1] : [VVMC_ShiftCount_enum <= VVMC_RollAveCount_enum]
    (junction 7) -> (junction 8) : {% Rolling Average
        |  VVMC_VehSpdRollAveRaw_kph = VVMC_VehSpdRollAveRaw_kph / VVMC_RollAveCount_enum;
        |
        |  % Rolling Average Counter
        |  VVMC_RollAveCount_enum++}
    (junction 35) -> (junction 5) : {VVMC_ShiftCount_enum++}
    (junction 6) -> (junction 36) : {% Rolling Average Sum
        |  VVMC_VehSpdRollAveRaw_kph = VVMC_VehSpdRollAveRaw_kph + VVMC_Memory_raw32[VVMC_ShiftCount_enum];
        |  }
    (junction 36) -> (junction 35)
    (junction 37) -> (junction 76) [order 1] : [VVMC_RollAveCount_enum == KVMC_VehSpdRollAveLevel_enum]
    (junction 76) -> (junction 47)
    (junction 37) -> (junction 60) [order 2]
    (junction 78) -> (junction 76)
    (junction 47) -> (junction 30) : {% Memory
        |  VVMC_Memory_raw32[VVMC_RollAveCount_enum] = VINP_VehSpeed_kph;
        |
        |  % Memory Shift Counter
        |  VVMC_ShiftCount_enum = ONE_INT;
        | }
    (junction 60) -> (junction 62) [order 1] : [VVMC_RollAveCount_enum > KVMC_VehSpdRollAveLevel_enum]
    (junction 60) -> (junction 39) [order 2]
    (junction 62) -> (junction 66) : {VVMC_MemoryShiftCount_enum = ONE_INT}
    (junction 30) -> (junction 48) [order 2]
    (junction 30) -> (junction 22) [order 1] : [VVMC_ShiftCount_enum <= VVMC_RollAveCount_enum]
    (junction 48) -> (junction 45) : {% Rolling Average
        |  VVMC_VehSpdRollAveRaw_kph = VVMC_VehSpdRollAveRaw_kph / VVMC_RollAveCount_enum;
        |
        |  % Memory Shift Counter
        |  VVMC_ShiftCount_enum = ONE_INT}
    (junction 14) -> (junction 30) : {VVMC_ShiftCount_enum++}
    (junction 22) -> (junction 25) : {% Rolling Average Sum
        |  VVMC_VehSpdRollAveRaw_kph = VVMC_VehSpdRollAveRaw_kph + VVMC_Memory_raw32[VVMC_ShiftCount_enum]}
    (junction 66) -> (junction 82) [order 2]
    (junction 66) -> (junction 69) [order 1] : [VVMC_MemoryShiftCount_enum < VVMC_RollAveCount_enum]
    (junction 82) -> (junction 80) : {VVMC_RollAveCount_enum = KVMC_VehSpdRollAveLevel_enum}
    (junction 73) -> (junction 66) : {VVMC_MemoryShiftCount_enum++}
    (junction 69) -> (junction 71) : {VVMC_Memory_raw32[VVMC_MemoryShiftCount_enum] =...
        |  VVMC_Memory_raw32[VVMC_RollAveCount_enum - KVMC_VehSpdRollAveLevel_enum + VVMC_MemoryShiftCount_enum]}
    (junction 25) -> (junction 14)
    (junction 71) -> (junction 73)
    (junction 80) -> (junction 78)
    (junction 45) -> (junction 39) [order 2]
    (junction 45) -> (junction 15) [order 1] : [VVMC_ShiftCount_enum < VVMC_RollAveCount_enum]
    (junction 41) -> (junction 45) : { VVMC_ShiftCount_enum++}
    (junction 15) -> (junction 38) : {% Gy Memory Shift
        |  VVMC_Memory_raw32[VVMC_ShiftCount_enum] = VVMC_Memory_raw32[VVMC_ShiftCount_enum + ONE_INT]}
    (junction 38) -> (junction 41)
  data: KVMC_VehSpdRollAveLevel_enum input uint8; VVMC_ShiftCount_enum local uint8; VVMC_RollAveCount_enum local uint8; VVMC_Memory_raw32 local single size=256; ZERO_FLOAT input single; ONE_INT input uint8; VINP_VehSpeed_kph input single; VVMC_MemoryShiftCount_enum local uint8; VVMC_VehSpdRollAveRaw_kph output single
